simulink model "Inverter_1ph_VSI_R2017a"  (R2017a)
settings: Solver=FixedStepAuto  StartTime=0.0  StopTime=1  MaxStep=1e-6  RelTol=1e-3  EnableMultiTasking=on
libraries: powerlib x10, simulink x4
settings Model: Creator=shaheb  LastModifiedBy=karpa
settings DataIOCC: LimitDataPoints=on  SaveFormat=Array  SignalLoggingSaveFormat=ModelDataLogs
settings OptimizationCC: ExpressionDepthLimit=2147483647  LifeSpan=inf
settings DebuggingCC: UnderspecifiedInitializationDetection=Classic  MergeDetectMultiDrivingBlocksExec=none  SolverPrmCheckMsg=warning  FcnCallInpInsideContextMsg=warning  StateNameClashWarn=warning  SFUnexpectedBacktrackingDiag=warning  SFNoUnconditionalDefaultTransitionDiag=warning
settings HardwareCC: ProdBitPerPointer=32  ProdBitPerSizeT=32  ProdBitPerPtrDiffT=32  ProdLargestAtomicFloat=None  ProdIntDivRoundTo=Undefined  ProdEndianess=Unspecified  ProdWordSize=32  ProdHWDeviceType=32-bit Generic
settings ModelReferenceCC: PropagateSignalLabelsOutOfModel=off
settings GRTTargetCC: TargetLangStandard=C89/C90 (ANSI)  CombineOutputUpdateFcns=off  GRTInterface=on
settings ConfigComp: CovMetricSettings=dw  CovHtmlReporting=on  CovSaveCumulativeToWorkspaceVar=on  CovSaveSingleToWorkspaceVar=on  CovExternalEMLEnable=off
settings SimscapeCC: SimscapeNormalizeSystem=off

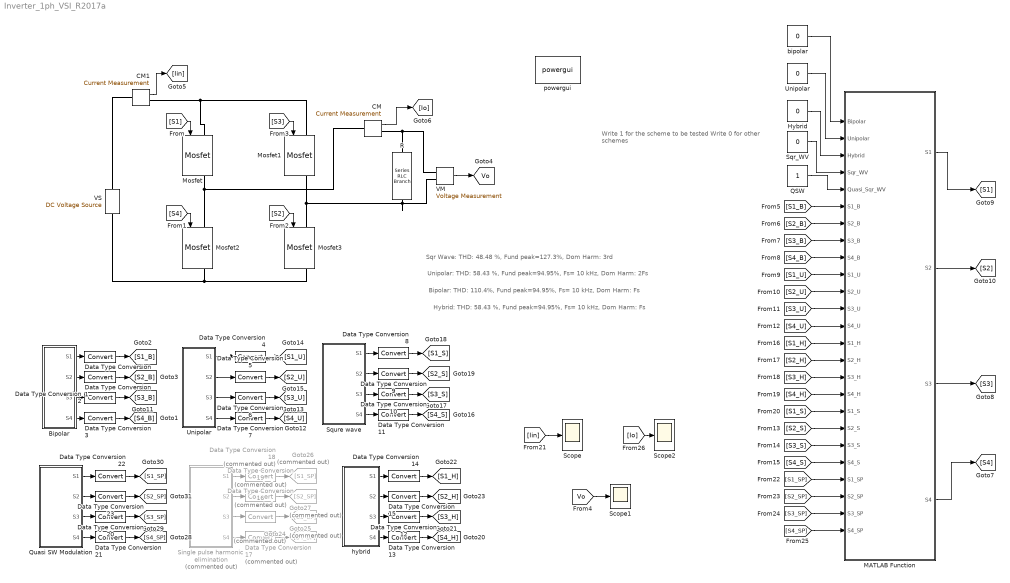
== system Inverter_1ph_VSI_R2017a ==
  note: Write 1 for the scheme to be tested
      | Write 0 for other schemes
  note: Hybrid: THD: 58.43 %, Fund peak=94.95%, Fs= 10 kHz, Dom Harm: Fs
  note: Bipolar: THD: 110.4%, Fund peak=94.95%, Fs= 10 kHz, Dom Harm: Fs
  note: Unipolar: THD: 58.43 %, Fund peak=94.95%, Fs= 10 kHz, Dom Harm: 2Fs
  note: Sqr Wave: THD: 48.48 %, Fund peak=127.3%, Dom Harm: 3rd
  Bipolar : Subsystem
  CM : powerlib/Measurements/Current Measurement  PhasorSimulation=off  OutputType=Complex  PSBequivalent=0
  CM1 : powerlib/Measurements/Current Measurement  PhasorSimulation=off  OutputType=Complex  PSBequivalent=0
  Data Type Conversion{,1..15,20..23} (20 alike) : DataTypeConversion
  Data Type Conversion{16..19} (4 alike) : DataTypeConversion  Commented=on
  Goto24 : Goto  Commented=on  GotoTag=S4_SP
  Goto25 : Goto  Commented=on  GotoTag=S3_SP
  Goto26 : Goto  Commented=on  GotoTag=S1_SP
  Goto27 : Goto  Commented=on  GotoTag=S2_SP
  Hybrid : Constant  Value=0
  MATLAB Function : MATLAB Function  TreatAsAtomicUnit=on
  Mosfet{,1..3} (4 alike) : powerlib/Power Electronics/Mosfet  Ron=0.02  Lon=0  Rd=0.001  Vfd=0.7  IC=0  Rs=1e5  Cs=inf  Measurements=on
  QSW : Constant
  Quasi SW Modulation : Subsystem
  R : powerlib/Elements/Series RLC Branch  LConnTagsString=__new0  RConnTagsString=__new0  BranchType=R  Resistance=40  Inductance=50e-3  SetiL0=off  InitialCurrent=0  Capacitance=500e-6  Setx0=off  InitialVoltage=0  Measurements=None
  Scope : Scope
  Scope1 : Scope
  Scope2 : Scope
  Single pulse harmonic elimination : Subsystem  Commented=on
  Sqr_WV : Constant  Value=0
  Squre wave : Subsystem
  Unipolar : Subsystem
  "Unipolar " : Constant  Value=0
  VM : powerlib/Measurements/Voltage Measurement  PhasorSimulation=off  OutputType=Complex  PSBequivalent=0
  VS : powerlib/Electrical Sources/DC Voltage Source  Amplitude=400  Measurements=None
  bipolar : Constant  Value=0
  hybrid : Subsystem
  powergui : powerlib/powergui  Priority=1  SimulationMode=Discrete  SampleTime=1e-6  frequency=60  Iterations=50  frequencyindice=0  Pbase=100e6  ErrMax=1e-4  UnitsV=kV  UnitsW=MW  buscounter=0  FunctionMessages=off  echomessages=off  EnableUseOfTLC=off  CurrentSourceSwitches=on  DisableSnubberDevices=off  DisableRonSwitches=off  DisableVfSwitches=off  DisplayEquations=off  AutomaticDiscreteSolvers=off  SolverType=Tustin  Interpol=off  ExternalGateDelay=off  methode=off  Ts=10  x0status=blocks  SPID=off  SwTol=0  HookPort=off  NonlinearTolerance=1e-4  nMaxIteration=100  ContinueOnMaxIteration=off  RestoreLinks=warning  ResistiveCurrentMeasurement=off  Frange=[0:2:500]  Ylog=off  Xlog=on  ShowGrid=off  save=off  variable=ZData  structure=vo  ZoomFFT=off  StartTime=0.3  cycles=20  DisplayStyle=1  fundamental=50  FreqAxis=off  MaxFrequency=25000  frequencyindicesteady=1  RmsSteady=1  display=off
  tag scope: Vo=global
  wires:
  [S1] -> Mosfet/1
  [S4] -> Mosfet2/1
  [S2] -> Mosfet3/1
  [S3] -> Mosfet1/1
  VM/1 -> [Vo]
  CM1/1 -> [Iin]
  CM/1 -> [Io]
  [Vo] -> Scope1/1
  Bipolar/1(S1) -> Data Type Conversion/1
  Bipolar/2(S2) -> Data Type Conversion1/1
  Bipolar/3(S3) -> Data Type Conversion2/1
  Bipolar/4(S4) -> Data Type Conversion3/1
  MATLAB Function/1(S1) -> [S1]
  MATLAB Function/2(S2) -> [S2]
  MATLAB Function/3(S3) -> [S3]
  MATLAB Function/4(S4) -> [S4]
  bipolar/1 -> MATLAB Function/1(Bipolar)
  "Unipolar "/1 -> MATLAB Function/2(Unipolar)
  Hybrid/1 -> MATLAB Function/3(Hybrid)
  Sqr_WV/1 -> MATLAB Function/4(Sqr_WV)
  [S1_B] -> MATLAB Function/6(S1_B)
  [S2_B] -> MATLAB Function/7(S2_B)
  [S3_B] -> MATLAB Function/8(S3_B)
  [S4_B] -> MATLAB Function/9(S4_B)
  Data Type Conversion/1 -> [S1_B]
  Data Type Conversion1/1 -> [S2_B]
  Data Type Conversion2/1 -> [S3_B]
  Data Type Conversion3/1 -> [S4_B]
  Data Type Conversion4/1 -> [S1_U]
  Data Type Conversion5/1 -> [S2_U]
  Data Type Conversion6/1 -> [S3_U]
  Data Type Conversion7/1 -> [S4_U]
  Unipolar/1(S1) -> Data Type Conversion4/1
  Unipolar/2(S2) -> Data Type Conversion5/1
  Unipolar/3(S3) -> Data Type Conversion6/1
  Unipolar/4(S4) -> Data Type Conversion7/1
  Data Type Conversion8/1 -> [S1_S]
  Data Type Conversion9/1 -> [S2_S]
  Data Type Conversion10/1 -> [S3_S]
  Data Type Conversion11/1 -> [S4_S]
  Squre wave/1(S1) -> Data Type Conversion8/1
  Squre wave/2(S2) -> Data Type Conversion9/1
  Squre wave/3(S3) -> Data Type Conversion10/1
  Squre wave/4(S4) -> Data Type Conversion11/1
  Data Type Conversion14/1 -> [S1_H]
  Data Type Conversion15/1 -> [S2_H]
  Data Type Conversion12/1 -> [S3_H]
  Data Type Conversion13/1 -> [S4_H]
  hybrid/1(S1) -> Data Type Conversion14/1
  hybrid/2(S2) -> Data Type Conversion15/1
  hybrid/3(S3) -> Data Type Conversion12/1
  hybrid/4(S4) -> Data Type Conversion13/1
  [S1_U] -> MATLAB Function/10(S1_U)
  [S2_U] -> MATLAB Function/11(S2_U)
  [S3_U] -> MATLAB Function/12(S3_U)
  [S4_U] -> MATLAB Function/13(S4_U)
  [S1_H] -> MATLAB Function/14(S1_H)
  [S4_H] -> MATLAB Function/17(S4_H)
  [S2_H] -> MATLAB Function/15(S2_H)
  [S2_S] -> MATLAB Function/19(S2_S)
  [S3_S] -> MATLAB Function/20(S3_S)
  [S4_S] -> MATLAB Function/21(S4_S)
  [S3_H] -> MATLAB Function/16(S3_H)
  [S1_S] -> MATLAB Function/18(S1_S)
  [Iin] -> Scope/1
  Single pulse harmonic elimination/4(S4) -> Data Type Conversion17/1
  Single pulse harmonic elimination/3(S3) -> Data Type Conversion16/1
  Single pulse harmonic elimination/2(S2) -> Data Type Conversion19/1
  Single pulse harmonic elimination/1(S1) -> Data Type Conversion18/1
  Data Type Conversion17/1 -> Goto24/1
  Data Type Conversion16/1 -> Goto25/1
  Data Type Conversion19/1 -> Goto27/1
  Data Type Conversion18/1 -> Goto26/1
  QSW/1 -> MATLAB Function/5(Quasi_Sqr_WV)
  [S1_SP] -> MATLAB Function/22(S1_SP)
  [S2_SP] -> MATLAB Function/23(S2_SP)
  [S3_SP] -> MATLAB Function/24(S3_SP)
  [S4_SP] -> MATLAB Function/25(S4_SP)
  [Io] -> Scope2/1
  Data Type Conversion22/1 -> [S1_SP]
  Data Type Conversion23/1 -> [S2_SP]
  Data Type Conversion20/1 -> [S3_SP]
  Data Type Conversion21/1 -> [S4_SP]
  Quasi SW Modulation/1(S1) -> Data Type Conversion22/1
  Quasi SW Modulation/2(S2) -> Data Type Conversion23/1
  Quasi SW Modulation/3(S3) -> Data Type Conversion20/1
  Quasi SW Modulation/4(S4) -> Data Type Conversion21/1
  connections:
  VM/LConn2 -- R/RConn1 -- Mosfet3/LConn1 -- Mosfet1/RConn1
  VS/LConn1 -- Mosfet3/RConn1 -- Mosfet2/RConn1
  CM/RConn1 -- VM/LConn1 -- R/LConn1
  CM/LConn1 -- Mosfet2/LConn1 -- Mosfet/RConn1
  VS/RConn1 -- CM1/LConn1
  CM1/RConn1 -- Mosfet1/LConn1 -- Mosfet/LConn1

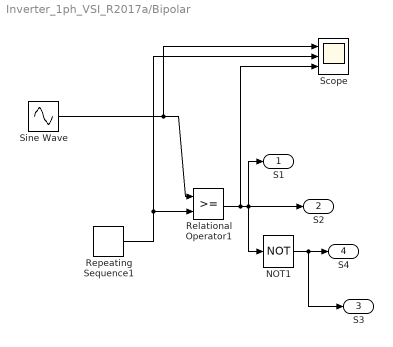
== system Inverter_1ph_VSI_R2017a/Bipolar ==
  NOT1 : Logic  Operator=NOT  AllPortsSameDT=off  OutDataTypeStr=boolean
  Relational Operator1 : RelationalOperator  OutDataTypeStr=boolean  RndMeth=Nearest
  Repeating Sequence1 : simulink/Sources/Repeating Sequence  rep_seq_t=[0 0.000025 0.00005 0.000075 0.0001]  rep_seq_y=[0 1 0 -1 0]
  Scope : Scope  NumInputPorts=3
  Sine Wave : Sin  Amplitude=.95  Frequency=2*pi*50  SampleTime=0
  S1 : Outport
  S2 : Outport  Port=2
  S3 : Outport  Port=3
  S4 : Outport  Port=4
  wires:
  Sine Wave/1 -> Scope/1, Relational Operator1/1
  Relational Operator1/1 -> Scope/3, S1/1, S2/1, NOT1/1
  NOT1/1 -> S3/1, S4/1
  Repeating Sequence1/1 -> Scope/2, Relational Operator1/2

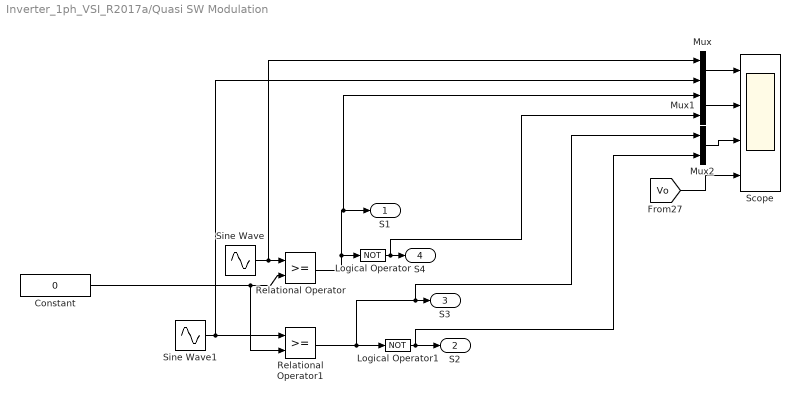
== system Inverter_1ph_VSI_R2017a/Quasi SW Modulation ==
  Constant : Constant  Value=0
  Logical Operator : Logic  Operator=NOT  AllPortsSameDT=off  OutDataTypeStr=boolean
  Logical Operator1 : Logic  Operator=NOT  AllPortsSameDT=off  OutDataTypeStr=boolean
  Mux : Mux  Inputs=2
  Mux1 : Mux  Inputs=2
  Mux2 : Mux  Inputs=2
  Relational Operator : RelationalOperator  OutDataTypeStr=boolean  RndMeth=Nearest
  Relational Operator1 : RelationalOperator  OutDataTypeStr=boolean  RndMeth=Nearest
  Scope : Scope  NumInputPorts=4
  Sine Wave : Sin  Amplitude=325  Frequency=314.157  SampleTime=0
  Sine Wave1 : Sin  Amplitude=325  Frequency=314.157  Phase=-pi*(1/3)  SampleTime=0
  S1 : Outport
  S2 : Outport  Port=2
  S3 : Outport  Port=3
  S4 : Outport  Port=4
  wires:
  Sine Wave1/1 -> Mux/2, Relational Operator1/1
  Constant/1 -> Relational Operator1/2, Relational Operator/2
  Sine Wave/1 -> Mux/1, Relational Operator/1
  Relational Operator1/1 -> Logical Operator1/1, Mux2/1, S3/1
  [Vo] -> Scope/4
  Mux/1 -> Scope/1
  Mux2/1 -> Scope/3
  Mux1/1 -> Scope/2
  Relational Operator/1 -> Mux1/1, S1/1, Logical Operator/1
  Logical Operator/1 -> Mux1/2, S4/1
  Logical Operator1/1 -> Mux2/2, S2/1

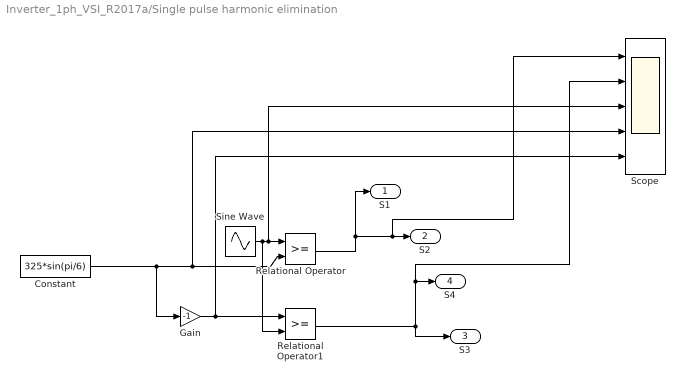
== system Inverter_1ph_VSI_R2017a/Single pulse harmonic elimination ==
  Constant : Constant  Value=325*sin(pi/6)
  Gain : Gain  Gain=-1
  Relational Operator : RelationalOperator  OutDataTypeStr=boolean  RndMeth=Nearest
  Relational Operator1 : RelationalOperator  OutDataTypeStr=boolean  RndMeth=Nearest
  Scope : Scope  NumInputPorts=5
  Sine Wave : Sin  Amplitude=325  Frequency=314.157  SampleTime=0
  S1 : Outport
  S2 : Outport  Port=2
  S3 : Outport  Port=3
  S4 : Outport  Port=4
  wires:
  Relational Operator1/1 -> S4/1, Scope/2, S3/1
  Relational Operator/1 -> S2/1, Scope/1, S1/1
  Sine Wave/1 -> Relational Operator1/2, Relational Operator/1, Scope/3
  Constant/1 -> Relational Operator/2, Scope/4, Gain/1
  Gain/1 -> Relational Operator1/1, Scope/5

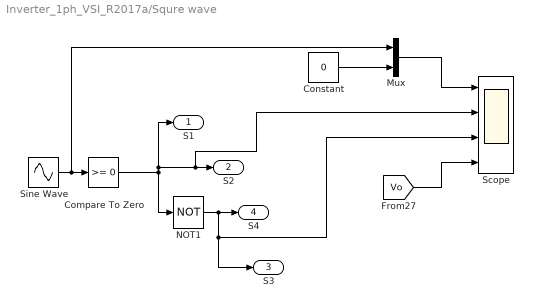
== system Inverter_1ph_VSI_R2017a/Squre wave ==
  Compare To Zero : simulink/Logic and Bit Operations/Compare To Zero  relop=>=  OutDataTypeStr=boolean
  Constant : Constant  Value=0
  Mux : Mux  Inputs=2
  NOT1 : Logic  Operator=NOT  AllPortsSameDT=off  OutDataTypeStr=boolean
  Scope : Scope  NumInputPorts=4
  Sine Wave : Sin  Amplitude=325  Frequency=314.157  SampleTime=0
  S1 : Outport
  S2 : Outport  Port=2
  S3 : Outport  Port=3
  S4 : Outport  Port=4
  wires:
  Sine Wave/1 -> Mux/1, Compare To Zero/1
  Compare To Zero/1 -> S1/1, Scope/2, S2/1, NOT1/1
  NOT1/1 -> Scope/3, S3/1, S4/1
  Constant/1 -> Mux/2
  Mux/1 -> Scope/1
  [Vo] -> Scope/4

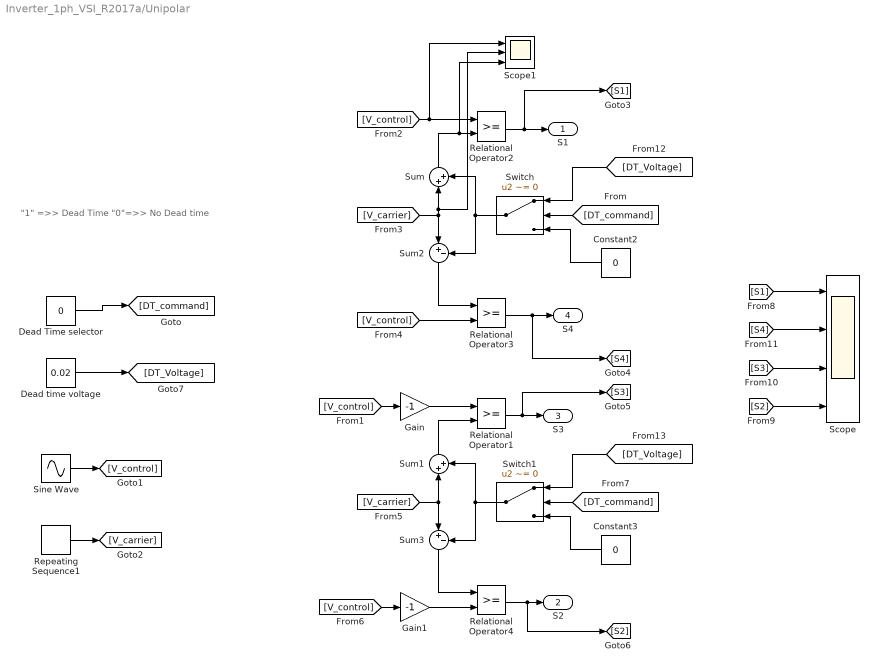
== system Inverter_1ph_VSI_R2017a/Unipolar ==
  note: "1" =>> Dead Time
      | "0"=>> No Dead time
  Constant2 : Constant  Value=0
  Constant3 : Constant  Value=0
  Dead Time selector : Constant  Value=0
  Dead time voltage : Constant  Value=0.02
  Gain : Gain  Gain=-1
  Gain1 : Gain  Gain=-1
  Relational Operator{1..4} (4 alike) : RelationalOperator  OutDataTypeStr=boolean  RndMeth=Nearest
  Repeating Sequence1 : simulink/Sources/Repeating Sequence  rep_seq_t=[0 0.000025 0.00005 0.000075 0.0001]  rep_seq_y=[0 1 0 -1 0]
  Scope : Scope  NumInputPorts=4
  Scope1 : Scope  NumInputPorts=3
  Sine Wave : Sin  Amplitude=.95  Frequency=2*pi*50  SampleTime=0
  Sum : Sum  Inputs=|++
  Sum1 : Sum  Inputs=|++
  Sum2 : Sum  Inputs=|+-
  Sum3 : Sum  Inputs=|+-
  Switch : Switch  Criteria=u2 ~= 0
  Switch1 : Switch  Criteria=u2 ~= 0
  S1 : Outport
  S2 : Outport  Port=2
  S3 : Outport  Port=3
  S4 : Outport  Port=4
  wires:
  [DT_Voltage] -> Switch/1
  Dead Time selector/1 -> [DT_command]
  Sine Wave/1 -> [V_control]
  Repeating Sequence1/1 -> [V_carrier]
  [V_carrier] -> Scope1/2, Sum/1, Sum2/1
  [V_control] -> Relational Operator3/2
  [DT_command] -> Switch/2
  Switch/1 -> Sum2/2, Sum/2
  Constant2/1 -> Switch/3
  [V_control] -> Scope1/1, Relational Operator2/1
  Sum/1 -> Scope1/3, Relational Operator2/2
  Sum2/1 -> Relational Operator3/1
  Relational Operator2/1 -> [S1], S1/1
  Relational Operator3/1 -> [S4], S4/1
  Switch1/1 -> Sum3/2, Sum1/2
  Relational Operator4/1 -> [S2], S2/1
  Sum1/1 -> Relational Operator1/2
  [V_carrier] -> Sum3/1, Sum1/1
  Relational Operator1/1 -> [S3], S3/1
  [V_control] -> Gain/1
  [V_control] -> Gain1/1
  Sum3/1 -> Relational Operator4/1
  Constant3/1 -> Switch1/3
  [DT_Voltage] -> Switch1/1
  [DT_command] -> Switch1/2
  Gain/1 -> Relational Operator1/1
  Gain1/1 -> Relational Operator4/2
  [S1] -> Scope/1
  [S3] -> Scope/3
  [S4] -> Scope/2
  [S2] -> Scope/4
  Dead time voltage/1 -> [DT_Voltage]

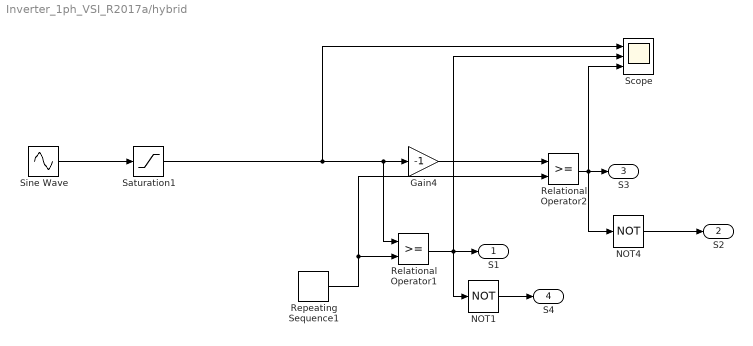
== system Inverter_1ph_VSI_R2017a/hybrid ==
  Gain4 : Gain  Gain=-1
  NOT1 : Logic  Operator=NOT  AllPortsSameDT=off  OutDataTypeStr=boolean
  NOT4 : Logic  Operator=NOT  AllPortsSameDT=off  OutDataTypeStr=boolean
  Relational Operator1 : RelationalOperator  OutDataTypeStr=boolean  RndMeth=Nearest
  Relational Operator2 : RelationalOperator  OutDataTypeStr=boolean  RndMeth=Nearest
  Repeating Sequence1 : simulink/Sources/Repeating Sequence  rep_seq_t="[0  0.00005 0.0001]"  rep_seq_y=[0 1 0]
  Saturation1 : Saturate  UpperLimit=1  LowerLimit=-1
  Scope : Scope  NumInputPorts=3
  Sine Wave : Sin  Amplitude=.95  Frequency=2*pi*50  SampleTime=0
  S1 : Outport
  S2 : Outport  Port=2
  S3 : Outport  Port=3
  S4 : Outport  Port=4
  wires:
  Sine Wave/1 -> Saturation1/1
  Saturation1/1 -> Scope/1, Relational Operator1/1, Gain4/1
  NOT4/1 -> S2/1
  Relational Operator2/1 -> Scope/3, S3/1, NOT4/1
  Gain4/1 -> Relational Operator2/1
  NOT1/1 -> S4/1
  Relational Operator1/1 -> Scope/2, NOT1/1, S1/1
  Repeating Sequence1/1 -> Relational Operator2/2, Relational Operator1/2

== matlab function Inverter_1ph_VSI_R2017a/MATLAB Function ==
  data: Bipolar input; S1 output; Unipolar input; Hybrid input; Sqr_WV input; Quasi_Sqr_WV input; S2 output; S3 output; S4 output; S1_B input; S2_B input; S3_B input; S4_B input; S1_U input; S2_U input; S3_U input; S4_U input; S1_H input; S2_H input; S3_H input; S4_H input; S1_S input; S2_S input; S3_S input; S4_S input; S1_SP input; S2_SP input; S3_SP input; S4_SP input
function [S1, S2, S3, S4]= fcn(Bipolar, Unipolar, Hybrid, Sqr_WV, Quasi_Sqr_WV, S1_B, S2_B, S3_B ,S4_B,S1_U, S2_U, S3_U ,S4_U, S1_H, S2_H, S3_H ,S4_H, S1_S, S2_S, S3_S ,S4_S,S1_SP, S2_SP, S3_SP ,S4_SP)
%#codegen

if Bipolar==1;
    S1=S1_B;
    S2=S2_B;
    S3=S3_B;
    S4=S4_B;
elseif Unipolar==1;
    S1=S1_U;
    S2=S2_U;
    S3=S3_U;
    S4=S4_U;
elseif Hybrid==1;
    S1=S1_H;
    S2=S2_H;
    S3=S3_H;
    S4=S4_H;
elseif Sqr_WV==1;
    S1=S1_S;
    S2=S2_S;
    S3=S3_S;
    S4=S4_S;
else Quasi_Sqr_WV=1;
    S1=S1_SP;
    S2=S2_SP;
    S3=S3_SP;
    S4=S4_SP;
     end
